simulink model "project2"  (Simulink 7.4)
settings: Solver=ode45  StartTime=0.0  StopTime=10.0  RelTol=1e-3
values from neighbouring files (symbols this model uses):
  A = [1 2; 3 4]    [control_system_project02.m]
  B = [0.4;0.3]    [control_system_project02.m]
  C = [1 0.4]    [control_system_project02.m]
  K = place(A,B,desired_controller_values)    [control_system_project02.m]
  L = place(A',C',desired_observer_values)'    [control_system_project02.m]
settings Model: Creator=Ashfaq  LastModifiedBy=Ashfaq

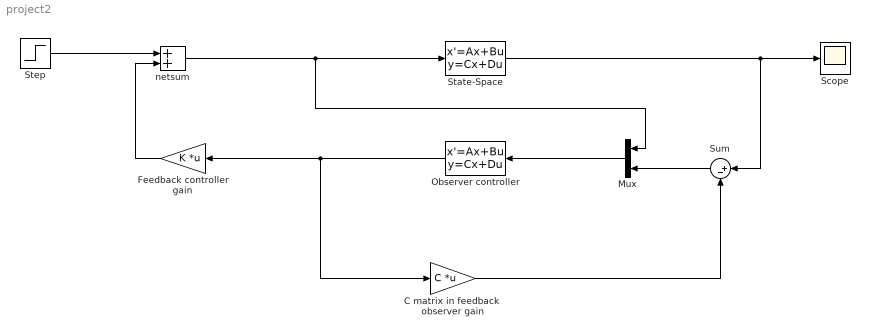
== system project2 ==
  C matrix in feedback  observer gain : Gain  Gain=C  Multiplication=Matrix(K*u)  ParameterDataType=fixdt(1, 16)  ParameterScaling=2^0  OutDataType=fixdt(1, 16)  OutScaling=2^0
  Feedback controller gain : Gain  Gain=K  Multiplication=Matrix(K*u)  ParameterDataType=fixdt(1, 16)  ParameterScaling=2^0  OutDataType=fixdt(1, 16)  OutScaling=2^0
  Mux : Mux  Inputs=2
  Observer controller : StateSpace  A=A  B=[B L]  C=[1 0;0 1]  D=[0 0;0 0]
  Scope : Scope
  State-Space : StateSpace
  Step : Step  SampleTime=0
  Sum : Sum  Inputs=|+-  OutDataType=fixdt(1, 16)  OutScaling=2^0
  netsum : Sum  Inputs=2  OutDataType=sfix(16)  OutScaling=2^0  SaturateOnIntegerOverflow=on  InputSameDT=on  OutDataTypeStr=Inherit: Same as first input
  wires:
  Step/1 -> netsum/1
  netsum/1 -> State-Space/1, Mux/1
  State-Space/1 -> Scope/1, Sum/1
  Sum/1 -> Mux/2
  C matrix in feedback  observer gain/1 -> Sum/2
  Mux/1 -> Observer controller/1
  Observer controller/1 -> Feedback controller gain/1, C matrix in feedback  observer gain/1
  Feedback controller gain/1 -> netsum/2
